simulink model "provaUML"  (R2022b)
settings: Solver=FixedStepAuto  StartTime=0.0  StopTime=100  FixedStep=1  RelTol=1e-3
values from neighbouring files (symbols this model uses):
  B = buttonPressInterval    [Excel2FileSim.m]    (also in buttonSim.m; excel3FileSim.m; excelSim.m; singleExec.m = 8)
  BD = 1    [buttonSim.m]
  TB = bcTimeInterval(j)    [Excel2FileSim.m]    (also in buttonSim.m; excel3FileSim.m; excelSim.m; singleExec.m = 2)
  TBD = 10    [buttonSim.m]
  TS = scannerTimeInterval(i)    [Excel2FileSim.m]    (also in buttonSim.m; excel3FileSim.m; excelSim.m; singleExec.m = 3)
  TSD = 10    [buttonSim.m]
libraries: simulink x2
settings Model: Creator=lolli  LastModifiedBy=lolli

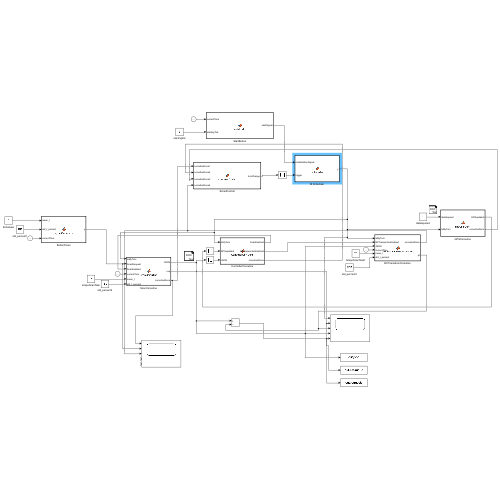
[thumbnail: Simulink's stored preview of the top-level diagram]
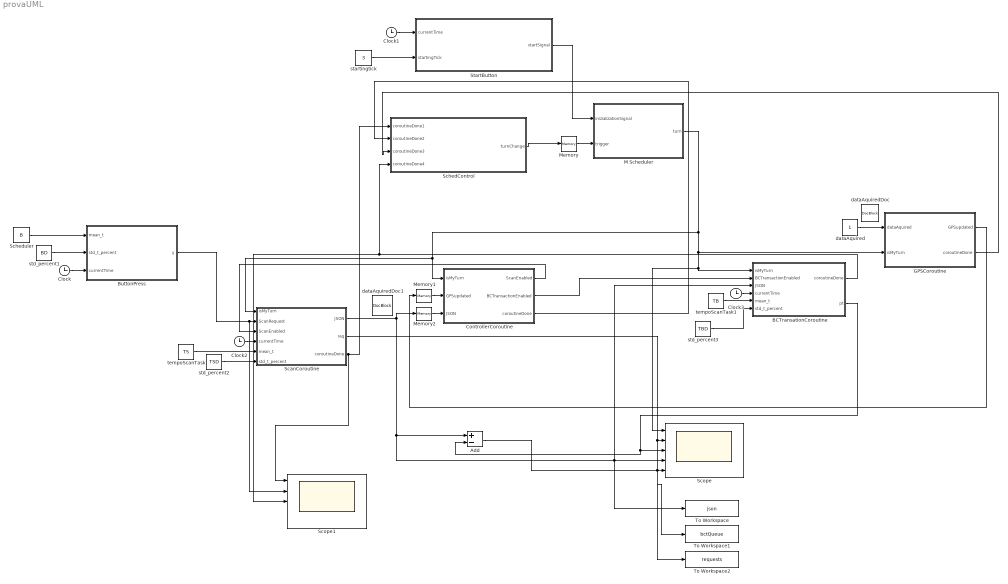
== system provaUML ==
  Add : Sum  Inputs=+-
  BCTransationCoroutine : MATLAB Function  TreatAsAtomicUnit=on
  ButtonPress : MATLAB Function  TreatAsAtomicUnit=on
  Clock{,1..3} (4 alike) : Clock
  ControllerCoroutine : MATLAB Function  TreatAsAtomicUnit=on
  GPSCoroutine : MATLAB Function  TreatAsAtomicUnit=on
  M Scheduler : MATLAB Function  TreatAsAtomicUnit=on
  Memory : Memory
  Memory1 : Memory
  Memory2 : Memory
  ScanCoroutine : MATLAB Function  TreatAsAtomicUnit=on
  SchedControl : MATLAB Function  TreatAsAtomicUnit=on
  Scheduler : Constant  Value=B
  Scope : Scope  NumInputPorts=5
  Scope1 : Scope  NumInputPorts=5
  StartButton : MATLAB Function  TreatAsAtomicUnit=on
  To Workspace : ToWorkspace  VariableName=json  SaveFormat=Timeseries  SampleTime=-1
  To Workspace1 : ToWorkspace  VariableName=bctQueue  SaveFormat=Timeseries  SampleTime=-1
  To Workspace2 : ToWorkspace  VariableName=requests  SaveFormat=Timeseries  SampleTime=-1
  dataAquired : Constant
  dataAquiredDoc : simulink/Model-Wide Utilities/DocBlock  DocumentType=Text
      content=|
      | Nel nostro caso il gps riesce sempre a ottenere i dati, se si vuole testare il caso in cui il gps fallisce mettere la costante a 0
  dataAquiredDoc1 : simulink/Model-Wide Utilities/DocBlock  DocumentType=Text
      content=|
      | Il json deve avere valori differenti non so come è da ragionare
  startingtick : Constant  Value=3
  std_percent1 : Constant  Value=BD
  std_percent2 : Constant  Value=TSD
  std_percent3 : Constant  Value=TBD
  tempoScanTask : Constant  Value=TS
  tempoScanTask1 : Constant  Value=TB
  wires:
  Clock/1 -> ButtonPress/3(currentTime)
  std_percent1/1 -> ButtonPress/2(std_t_percent)
  Scheduler/1 -> ButtonPress/1(mean_t)
  M Scheduler/1(turn) -> Scope/1, BCTransationCoroutine/1(isMyTurn), GPSCoroutine/2(isMyTurn), ControllerCoroutine/1(isMyTurn), ScanCoroutine/1(isMyTurn)
  GPSCoroutine/1(GPSupdated) -> Memory1/1
  ControllerCoroutine/1(ScanEnabled) -> ScanCoroutine/3(ScanEnabled)
  tempoScanTask/1 -> ScanCoroutine/5(mean_t)
  Clock2/1 -> ScanCoroutine/4(currentTime)
  dataAquired/1 -> GPSCoroutine/1(dataAquired)
  Memory/1 -> M Scheduler/2(trigger)
  SchedControl/1(turnChange) -> Memory/1
  ScanCoroutine/3(coroutineDone) -> Scope1/1, SchedControl/1(coroutineDone1)
  StartButton/1(startSignal) -> M Scheduler/1(inizializationSignal)
  Clock1/1 -> StartButton/1(currentTime)
  startingtick/1 -> StartButton/2(startingTick)
  ControllerCoroutine/3(coroutineDone) -> SchedControl/2(coroutineDone2)
  GPSCoroutine/2(coroutineDone) -> SchedControl/3(coroutineDone3)
  Memory1/1 -> ControllerCoroutine/2(GPSupdated)
  ScanCoroutine/1(JSON) -> Memory2/1, BCTransationCoroutine/3(JSON), Scope/4, To Workspace/1, Add/1
  tempoScanTask1/1 -> BCTransationCoroutine/5(mean_t)
  Clock3/1 -> BCTransationCoroutine/4(currentTime)
  ControllerCoroutine/2(BCTransactionEnabled) -> BCTransationCoroutine/2(BCTransactionEnabled)
  Memory2/1 -> ControllerCoroutine/3(JSON)
  BCTransationCoroutine/1(coroutineDone) -> Scope1/3, SchedControl/4(coroutineDone4)
  ButtonPress/1(y) -> Scope1/2, ScanCoroutine/2(ScanRequest)
  BCTransationCoroutine/2(pt) -> Add/2, Scope/3
  Add/1 -> To Workspace1/1, Scope/5
  ScanCoroutine/2(req) -> To Workspace2/1, Scope/2
  std_percent2/1 -> ScanCoroutine/6(std_t_percent)
  std_percent3/1 -> BCTransationCoroutine/6(std_t_percent)

== matlab function provaUML/GPSCoroutine ==
  data: dataAquired input; GPSupdated output; isMyTurn input; coroutineDone output
function [GPSupdated, coroutineDone] = gpsCoroutine(dataAquired, isMyTurn)

    persistent state;
    
    if isempty(state)
        state = 0;
    end
    
    % se non è il turno della coroutine
    if isMyTurn == 0
 
        if dataAquired == 1
            state = 1;  % GPS update completato
        end

        coroutineDone = 1;  % Coroutine completata
    else 
        coroutineDone = 0;  % Coroutine non completata
    end
    
%     if isMyTurn == 0 && state == 1
%         coroutineDone = 1;  % Coroutine completata
%     else
%         coroutineDone = 0;  % Coroutine non completata
%     end


    GPSupdated = state;
end

== matlab function provaUML/ButtonPress ==
  data: mean_t input; std_t_percent input; y output; currentTime input
function y = signalGenerator(mean_t, std_t_percent, currentTime)
    % derivazione standard in percentuale
    std_t = (mean_t * std_t_percent) / 100;

    persistent nextTriggerTime

    % inizializza triggerTime
    if isempty(nextTriggerTime)
        nextTriggerTime = mean_t + std_t * randn; % rende funzione stocastica
    end

    % controllo se generare il segnale
    if currentTime >= nextTriggerTime
        y = 1; 
        nextTriggerTime = currentTime + mean_t + std_t * randn;
    else
        y = 0; % No signal output
    end
end

== matlab function provaUML/ControllerCoroutine ==
  data: isMyTurn input; GPSupdated input; ScanEnabled output; BCTransactionEnabled output; coroutineDone output; JSON input
function [ScanEnabled, BCTransactionEnabled, coroutineDone] = ControllerCoroutine(isMyTurn, GPSupdated, JSON)
    % ScanEnabled: indica se la scansione è abilitata (1 o 0)
    % BCTransactionEnabled: indica se la transazione BC è abilitata (1 o 0)

    % mantengono lo stato della coroutine
    persistent scanState bctState;

    % inizializzazione variabili
    if isempty(scanState)
        scanState = 0;
    end
    if isempty(bctState)
        bctState = 0;
    end

    if isMyTurn == 1
        if JSON > 0
            bctState = 1;  % abilita la transazione BC
        else
            bctState = 0;  % disabilita la transazione BC
        end
    end

    if isMyTurn == 1
        if GPSupdated == 1
            scanState = 1;  % abilita la scansione
            coroutineDone = 1;  % coroutine completata
        else
            scanState = 0;  % disabilita la scansione
            coroutineDone = 1;  % coroutine completata
        end
    else
        coroutineDone = 0;  % coroutine non completata
    end

    % ste output
    ScanEnabled = scanState;
    BCTransactionEnabled = bctState;
end

== matlab function provaUML/M Scheduler ==
  data: inizializationSignal input; turn output; trigger input
function turn = scheduler(inizializationSignal, trigger)

    persistent currentIndex prevTrigger;
    
    % inizializzazione variabili persistenti
    if isempty(currentIndex)
        currentIndex = -1;  
    end
    if isempty(prevTrigger)
        prevTrigger = -1;  
    end

    if inizializationSignal == 1
        currentIndex = 0;
        prevTrigger = 0;
    end

    % controllo rising edge input
    if prevTrigger == 0 && trigger == 1
        % incrementa l'indice ciclicamente (0, 1, 2, 3, poi ripeti)
        currentIndex = mod(currentIndex + 1, 4);
    end

    % salva vecchio valore
    prevTrigger = trigger;
    turn = currentIndex;
end

== matlab function provaUML/ScanCoroutine ==
  data: isMyTurn input; ScanRequest input; ScanEnabled input; currentTime input; mean_t input; std_t_percent input; JSON output; req output; coroutineDone output
function [JSON, req,coroutineDone] = ScanCoroutine(isMyTurn, ScanRequest, ScanEnabled, currentTime, mean_t, std_t_percent)
    persistent state startTime on requests state2 t;

    % inizializza varioabili
    if isempty(state)
        state = 0;
        startTime = 0;
        on = 0;
        requests = 0;
        state2 = 0;
        t = mean_t;
    end

    if ScanRequest == 1
        requests = requests + 1;
    end

    if isMyTurn == 2 && requests == 0
        JSON = state;
        req = requests;
        coroutineDone = 1;
        return;
    end

    % inizio conteggio tempo coroutine
    if ScanEnabled == 1 && on == 0
        % salva tempo iniziale
        startTime = currentTime;
        % imposta durata stocastica della funzione
        std_t = (mean_t * std_t_percent) / 100;
        t = mean_t + std_t * randn; 
        on = 1;  
    end
    
    % tempo completato
    if currentTime >= startTime + t && on == 1 && isMyTurn == 2
        state = state + 1;  % jeson creato (+1)
        state2 = 1;
    end
    
    JSON = state;
    req = requests;

    % segnala fine della coroutine se terminata
    if isMyTurn == 2 && state2 == 1
        coroutineDone = 1;  
        on = 0;             
        requests = requests -1;
        state2 = 0;          
    else
        coroutineDone = 0;  
    end
end

== matlab function provaUML/SchedControl ==
  data: coroutineDone1 input; turnChange output; coroutineDone2 input; coroutineDone3 input; coroutineDone4 input
function turnChange = schedulerControl(coroutineDone1, coroutineDone2, coroutineDone3, coroutineDone4)

    persistent prevCoroutineDone1 prevCoroutineDone2 prevCoroutineDone3 prevCoroutineDone4 turnInProgress;

    % inizializza variabili persistenti
    if isempty(prevCoroutineDone1)
        prevCoroutineDone1 = 0;
        prevCoroutineDone2 = 0;
        prevCoroutineDone3 = 0;
        prevCoroutineDone4 = 0;
        turnInProgress = 0;  % stato x reset
    end

    if turnInProgress == 1
        turnChange = 0;
        turnInProgress = 0;  % reset x 1 tick
        return;
    end

    % controllo rising edge
    if (coroutineDone1 == 1 && prevCoroutineDone1 == 0) || ...
       (coroutineDone2 == 1 && prevCoroutineDone2 == 0) || ...
       (coroutineDone3 == 1 && prevCoroutineDone3 == 0) || ...
       (coroutineDone4 == 1 && prevCoroutineDone4 == 0)
        turnChange = 1;
        turnInProgress = 1;
    else
        turnChange = 0;
    end

    % aggiorna valori
    prevCoroutineDone1 = coroutineDone1;
    prevCoroutineDone2 = coroutineDone2;
    prevCoroutineDone3 = coroutineDone3;
    prevCoroutineDone4 = coroutineDone4;
end

== matlab function provaUML/StartButton ==
  data: currentTime input; startSignal output; startingTick input
function startSignal = Inizializator(currentTime, startingTick)
    startSignal = 0;
    if currentTime == startingTick
        startSignal = 1;  % inizia simulazione dopo tempo startingTick
    end
end

== matlab function provaUML/BCTransationCoroutine ==
  data: isMyTurn input; BCTransactionEnabled input; JSON input; currentTime input; mean_t input; coroutineDone output; pt output; std_t_percent input
function [coroutineDone, pt] = BCTransactionCoroutine(isMyTurn, BCTransactionEnabled, JSON, currentTime, mean_t, std_t_percent)

    persistent state startTime on processedTransactions t;

    % inizializza variabili persistenti
    if isempty(state)
        state = 0;
        startTime = 0;
        on = 0;
        processedTransactions = 0;  % transazioni già elaborate
        t = mean_t;
    end

    % se JSON è 0 o BCTransactionEnabled è 0, non eseguire nessuna transazione
    if isMyTurn == 3 && (JSON == 0 || BCTransactionEnabled == 0)
        coroutineDone = 1;
        state = 0;  % reset
        on = 0;     
        pt = -1;
        return;
    end

    % se ci sono nuove transazioni da eseguire (JSON > processedTransactions)
    if isMyTurn == 3 && JSON > processedTransactions && BCTransactionEnabled == 1
        % init conteggio
        if state == 0 && on == 0
            startTime = currentTime; % salva tempo iniziale per il conteggio
            on = 1;  
            % imposta durata stocastica della funzione
            std_t = (mean_t * std_t_percent) / 100;
            t = mean_t + std_t * randn; 
        end

        if currentTime >= startTime + t && on == 1
            state = 1;  % stato completato
        end
    end

    % controllo fine coroutine
    if isMyTurn == 3 && state == 1
        coroutineDone = 1;  
        processedTransactions = processedTransactions + 1;  % aggiorna transazioni 
        state = 0;  
        on = 0;     
    else
        coroutineDone = 0;  
    end

    pt = processedTransactions;
end
